simulink model "TV_Rev2_DynTest_SIMULINK"  (R2021a)
settings: Solver=FixedStepAuto  StartTime=0.0  StopTime=40  FixedStep=0.01  RelTol=1e-3
values from neighbouring files (symbols this model uses):
  Delta11T = xlsread('TV Dynamic Test data_EXCEL.xlsx', 'Steering','L2:L55' )    [TorqueVectoring_Rev2_Parameters_MATLAB.m]
  Delta12T = xlsread('TV Dynamic Test data_EXCEL.xlsx', 'Steering','M2:M55' )    [TorqueVectoring_Rev2_Parameters_MATLAB.m]
  DeltaT = xlsread('TV Dynamic Test data_EXCEL.xlsx', 'Steering','K2:K55' )    [TorqueVectoring_Rev2_Parameters_MATLAB.m]
  Tmaxf = 250    [TorqueVectoring_Rev2_Parameters_MATLAB.m]
  Tmaxr = 250    [TorqueVectoring_Rev2_Parameters_MATLAB.m]
undefined symbols (not defined in the file or in its folder): sigbuilder_block
libraries: simulink_extras x2
settings Model: Creator=CptBrownPants  LastModifiedBy=Pickett
settings SolverCC: AlgebraicLoopSolver=TrustRegion
settings OptimizationCC: DefaultParameterBehavior=Inlined  EnhancedBackFolding=on  PassReuseOutputArgsAs=Individual arguments  ZeroExternalMemoryAtStartup=off  ZeroInternalMemoryAtStartup=off  InitFltsAndDblsToZero=on  MaxStackSize=2048  OptimizeBlockOrder=speed  DifferentSizesBufferReuse=on  OptimizationCustomize=off  EfficientTunableParamExpr=on
settings DebuggingCC: ParameterTunabilityLossMsg=error  SFMachineParentedDataDiag=warning
settings HardwareCC: ProdBitPerPointer=32  ProdBitPerSizeT=32  ProdBitPerPtrDiffT=32  ProdLargestAtomicInteger=Long  ProdLargestAtomicFloat=Double  ProdEndianess=BigEndian  ProdWordSize=32  ProdHWDeviceType=Freescale->32-bit PowerPC
settings SFSimCC: MATLABDynamicMemAlloc=off
settings RTWCC: Description=Create UserLibraries for MoTeC M1 Build  SystemTargetFile=MoTeC.tlc  GenCodeOnly=on  TemplateMakefile=MoTeCUserlibMakefile.tmf  PostCodeGenCommand=MoTeCUtil.m1_post_process(buildInfo)
settings CodeAppCC: ForceParamTrailComments=on  IgnoreCustomStorageClasses=off  OperatorAnnotations=on  SimulinkDataObjDesc=on  SFDataObjDesc=on  InsertBlockDesc=on
settings STFCustomTargetCC: TargetLangStandard=C99 (ISO)  MultiwordLength=256  GenerateSampleERTMain=on  CombineOutputUpdateFcns=on  ERTCustomFileBanners=on  SupportContinuousTime=off  SupportNonInlinedSFcns=off  RemoveResetFunc=on  MATLABClassNameForMDSCustomization=Simulink.SoftwareTarget.ERTCustomization  GRTInterface=off  UseToolchainInfoCompliant=off  SystemTargetFile=MoTeC.tlc
settings ERTTargetCC: TargetLangStandard=C99 (ISO)  GenerateSampleERTMain=on  ParMdlRefBuildCompliant=off  CompOptLevelCompliant=off  ConcurrentExecutionCompliant=off  ModelStepFunctionPrototypeControlCompliant=off  CPPClassGenCompliant=off  UseToolchainInfoCompliant=off  InlinedParameterPlacement=NonHierarchical  ERTCustomFileTemplate=MoTeCFileProcess.tlc  EnableUserReplacementTypes=on

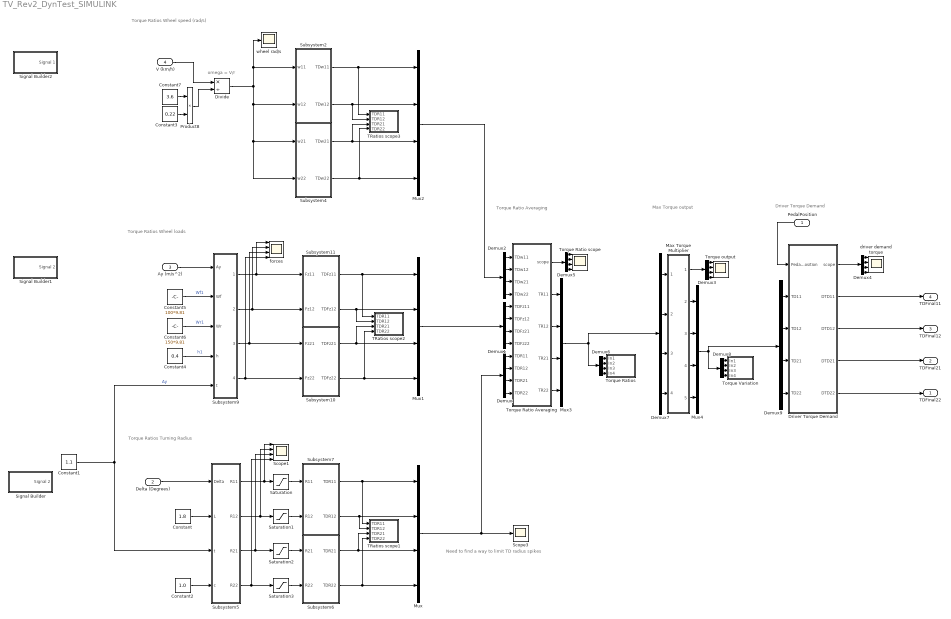
== system TV_Rev2_DynTest_SIMULINK ==
  note: Driver Torque Demand
  note: Max Torque output
  note: Torque Ratio Averaging
  note: Need to find a way to limit TD radius spikes
  note: Torque Ratios Wheel speed (rad/s)
  note: Torque Ratios Wheel loads
  note: Torque Ratios Turning Radius
  note: omega = V/r
  PedalPosition : Inport
  Delta (Degrees) : Inport  Port=2
  Ay (m/s^2) : Inport  Port=3
  V (km/h) : Inport  Port=4
  Constant : Constant  Value=1.8
  Constant1 : Constant  Value=1.1
  Constant2 : Constant  Value=1.0
  Constant3 : Constant  Value=0.22
  Constant4 : Constant  Value=0.4
  Constant5 : Constant  Value=100*9.81
  Constant6 : Constant  Value=150*9.81
  Constant7 : Constant  Value=3.6
  Demux{,1..9} (10 alike) : Demux
  Divide : Product  Inputs=*/
  Driver Torque Demand : Subsystem
  Max Torque Multiplier : Subsystem
  Mux{,1..4} (5 alike) : Mux
  Product8 : Product
  Saturation{,1..3} (4 alike) : Saturate  UpperLimit=100  LowerLimit=-100
  Scope1 : Scope  NumInputPorts=4
  Scope3 : Scope
  Signal Builder : Subsystem  Tag=STV Subsys  LoadFcn=sigbuilder_block('load');  StartFcn=sigbuilder_block('start');  StopFcn=sigbuilder_block('stop');  ClipboardFcn=sigbuilder_block('clipboard');  mask(Sigbuilder block){tuvar=[0:10]}
      mask help: Simulink:masks:SigbuilderBlock_MD
      mask init:
      | if ~strcmp(get_param(bdroot(gcbh),'SimulationStatus'),'stopped') tuvar = sigbuilder_block('maskInit'); end
      settings: CopyFcn=sigbuilder_block('copy');  DeleteFcn=sigbuilder_block('delete');  ModelCloseFcn=sigbuilder_block('modelClose');  PreSaveFcn=sigbuilder_block('preSave');  PauseFcn=sigbuilder_block('pause');  ContinueFcn=sigbuilder_block('continue');  NameChangeFcn=sigbuilder_block('namechange');  OpenFcn=sigbuilder_block('open',[143 201 550 400 ]);  CloseFcn=sigbuilder_block('close');
      mask Display: plot(0, 0, 100, 100,[2, 2, 32, 32, 2], [68, 8, 8, 68, 68],[32, 2], [38, 38], [32, 19, 2],[53, 60, 44], [32, 17, 17, 2],[16, 16, 31, 31]);txt = getActiveGroup(gcbh);text(2, 100, txt,'verticalAlignment', 'top');
  Signal Builder1 : Subsystem  Tag=STV Subsys  LoadFcn=sigbuilder_block('load');  StartFcn=sigbuilder_block('start');  StopFcn=sigbuilder_block('stop');  ClipboardFcn=sigbuilder_block('clipboard');  mask(Sigbuilder block){tuvar=[0:10]}
      mask help: Simulink:masks:SigbuilderBlock_MD
      mask init:
      | if ~strcmp(get_param(bdroot(gcbh),'SimulationStatus'),'stopped') tuvar = sigbuilder_block('maskInit'); end
      settings: CopyFcn=sigbuilder_block('copy');  DeleteFcn=sigbuilder_block('delete');  ModelCloseFcn=sigbuilder_block('modelClose');  PreSaveFcn=sigbuilder_block('preSave');  PauseFcn=sigbuilder_block('pause');  ContinueFcn=sigbuilder_block('continue');  NameChangeFcn=sigbuilder_block('namechange');  OpenFcn=sigbuilder_block('open',[437.6 199.2 550.4 400 ]);  CloseFcn=sigbuilder_block('close');
      mask Display: plot(0, 0, 100, 100,[2, 2, 32, 32, 2], [68, 8, 8, 68, 68],[32, 2], [38, 38], [32, 19, 2],[53, 60, 44], [32, 17, 17, 2],[16, 16, 31, 31]);txt = getActiveGroup(gcbh);text(2, 100, txt,'verticalAlignment', 'top');
  Signal Builder2 : Subsystem  Tag=STV Subsys  LoadFcn=sigbuilder_block('load');  StartFcn=sigbuilder_block('start');  StopFcn=sigbuilder_block('stop');  ClipboardFcn=sigbuilder_block('clipboard');  mask(Sigbuilder block){tuvar=[0:10]}
      mask help: Simulink:masks:SigbuilderBlock_MD
      mask init:
      | if ~strcmp(get_param(bdroot(gcbh),'SimulationStatus'),'stopped') tuvar = sigbuilder_block('maskInit'); end
      settings: CopyFcn=sigbuilder_block('copy');  DeleteFcn=sigbuilder_block('delete');  ModelCloseFcn=sigbuilder_block('modelClose');  PreSaveFcn=sigbuilder_block('preSave');  PauseFcn=sigbuilder_block('pause');  ContinueFcn=sigbuilder_block('continue');  NameChangeFcn=sigbuilder_block('namechange');  OpenFcn=sigbuilder_block('open',[437.6 199.2 550.4 400 ]);  CloseFcn=sigbuilder_block('close');
      mask Display: plot(0, 0, 100, 100,[2, 2, 32, 32, 2], [68, 8, 8, 68, 68],[32, 2], [38, 38], [32, 19, 2],[53, 60, 44], [32, 17, 17, 2],[16, 16, 31, 31]);txt = getActiveGroup(gcbh);text(2, 100, txt,'verticalAlignment', 'top');
  Subsystem10 : Subsystem
  Subsystem11 : Subsystem
  Subsystem2 : Subsystem
  Subsystem4 : Subsystem
  Subsystem5 : Subsystem
  Subsystem6 : Subsystem
  Subsystem7 : Subsystem
  Subsystem9 : Subsystem
  TRatios scope1 : Subsystem
  TRatios scope2 : Subsystem
  TRatios scope3 : Subsystem
  Torque Ratio Averaging : Subsystem
  Torque Ratio scope : Scope  NumInputPorts=4
  "Torque Ratios " : Subsystem
  Torque Variation : Subsystem
  Torque output : Scope  NumInputPorts=4
  driver demand torque : Scope  NumInputPorts=4
  forces : Scope  NumInputPorts=4
  wheel rad/s : Scope
  TDFinal22 : Outport
  TDFinal21 : Outport  Port=2
  TDFinal12 : Outport  Port=3
  TDFinal11 : Outport  Port=4
  wires:
  Subsystem2/2(TDw12) -> Mux2/2, TRatios scope3/2(TDR12)
  Subsystem2/1(TDw11) -> Mux2/1, TRatios scope3/1(TDR11)
  Subsystem4/2(TDw22) -> Mux2/4, TRatios scope3/4(TDR22)
  Subsystem4/1(TDw21) -> Mux2/3, TRatios scope3/3(TDR21)
  Subsystem7/2(TDR12) -> Mux/2, TRatios scope1/2(TDR12)
  Subsystem7/1(TDR11) -> Mux/1, TRatios scope1/1(TDR11)
  Subsystem6/2(TDR22) -> Mux/4, TRatios scope1/4(TDR22)
  Subsystem6/1(TDR21) -> Mux/3, TRatios scope1/3(TDR21)
  Subsystem5/1(R11) -> Scope1/1, Saturation/1
  Saturation/1 -> Subsystem7/1(R11)
  Subsystem5/2(R12) -> Scope1/2, Saturation1/1
  Subsystem5/4(R22) -> Saturation3/1, Scope1/4
  Subsystem5/3(R21) -> Saturation2/1, Scope1/3
  Constant1/1 -> Subsystem5/3(t), Subsystem9/5(t)  "Ay"
  Constant/1 -> Subsystem5/2(L)
  Saturation1/1 -> Subsystem7/2(R12)
  Constant2/1 -> Subsystem5/4(c)
  Saturation2/1 -> Subsystem6/1(R21)
  Saturation3/1 -> Subsystem6/2(R22)
  Subsystem9/2(Fz12) -> forces/2, Subsystem11/2(Fz12)
  Subsystem9/3(Fz21) -> forces/3, Subsystem10/1(Fz21)
  Constant4/1 -> Subsystem9/4(h)  "h1"
  Subsystem9/1(Fz11) -> Subsystem11/1(Fz11), forces/1
  Constant6/1 -> Subsystem9/3(Wr)  "Wr1"
  Subsystem9/4(Fz22) -> Subsystem10/2(Fz22), forces/4
  Constant5/1 -> Subsystem9/2(Wf)  "Wf1"
  Divide/1 -> wheel rad/s/1, Subsystem2/1(w11), Subsystem4/2(w22), Subsystem4/1(w21), Subsystem2/2(w12)
  Constant3/1 -> Product8/2
  Constant7/1 -> Product8/1
  Product8/1 -> Divide/2
  Mux/1 -> Demux/1, Scope3/1
  Demux/1 -> Torque Ratio Averaging/9(TDR11)
  Demux/2 -> Torque Ratio Averaging/10(TDR12)
  Demux/3 -> Torque Ratio Averaging/11(TDR21)
  Demux/4 -> Torque Ratio Averaging/12(TDR22)
  Subsystem10/1(TDFz21) -> Mux1/3, TRatios scope2/3(TDR21)
  Subsystem10/2(TDFz22) -> Mux1/4, TRatios scope2/4(TDR22)
  Subsystem11/2(TDFz12) -> Mux1/2, TRatios scope2/2(TDR12)
  Subsystem11/1(TDFz11) -> Mux1/1, TRatios scope2/1(TDR11)
  Demux1/1 -> Torque Ratio Averaging/5(TDFz11)
  Demux1/2 -> Torque Ratio Averaging/6(TDFz12)
  Demux1/3 -> Torque Ratio Averaging/7(TDFz21)
  Demux1/4 -> Torque Ratio Averaging/8(TDFz22)
  Mux1/1 -> Demux1/1
  Demux2/1 -> Torque Ratio Averaging/1(TDw11)
  Demux2/2 -> Torque Ratio Averaging/2(TDw12)
  Demux2/3 -> Torque Ratio Averaging/3(TDw21)
  Demux2/4 -> Torque Ratio Averaging/4(TDw22)
  Mux2/1 -> Demux2/1
  Demux3/2 -> Torque output/2
  Demux3/3 -> Torque output/3
  Demux3/4 -> Torque output/4
  Demux3/1 -> Torque output/1
  Demux4/1 -> driver demand torque/1
  Demux4/2 -> driver demand torque/2
  Demux4/3 -> driver demand torque/3
  Demux4/4 -> driver demand torque/4
  Driver Torque Demand/2(DTD11) -> TDFinal11/1
  Driver Torque Demand/3(DTD12) -> TDFinal12/1
  Driver Torque Demand/4(DTD21) -> TDFinal21/1
  Driver Torque Demand/5(DTD22) -> TDFinal22/1
  Max Torque Multiplier/1(scope) -> Demux3/1
  Driver Torque Demand/1(scope) -> Demux4/1
  Demux5/1 -> Torque Ratio scope/1
  Demux5/4 -> Torque Ratio scope/4
  Demux5/3 -> Torque Ratio scope/3
  Demux5/2 -> Torque Ratio scope/2
  Torque Ratio Averaging/1(scope) -> Demux5/1
  Torque Ratio Averaging/2(TR11) -> Mux3/1
  Torque Ratio Averaging/3(TR12) -> Mux3/2
  Torque Ratio Averaging/4(TR21) -> Mux3/3
  Torque Ratio Averaging/5(TR22) -> Mux3/4
  Demux6/3 -> "Torque Ratios "/3(In3)
  Demux6/1 -> "Torque Ratios "/1(In1)
  Demux6/2 -> "Torque Ratios "/2(In2)
  Demux6/4 -> "Torque Ratios "/4(In4)
  Mux3/1 -> Demux7/1, Demux6/1
  Demux7/1 -> Max Torque Multiplier/1(TR11)
  Demux7/2 -> Max Torque Multiplier/2(TR12)
  Demux7/3 -> Max Torque Multiplier/3(TR21)
  Demux7/4 -> Max Torque Multiplier/4(TR22)
  Max Torque Multiplier/2(TD11) -> Mux4/1
  Max Torque Multiplier/3(TD12) -> Mux4/2
  Max Torque Multiplier/4(TD21) -> Mux4/3
  Max Torque Multiplier/5(TD22) -> Mux4/4
  Demux8/4 -> Torque Variation/4(In4)
  Demux8/2 -> Torque Variation/2(In2)
  Demux8/1 -> Torque Variation/1(In1)
  Demux8/3 -> Torque Variation/3(In3)
  Mux4/1 -> Demux9/1, Demux8/1
  Demux9/1 -> Driver Torque Demand/2(TD11)
  Demux9/2 -> Driver Torque Demand/3(TD12)
  Demux9/3 -> Driver Torque Demand/4(TD21)
  Demux9/4 -> Driver Torque Demand/5(TD22)
  Delta (Degrees)/1 -> Subsystem5/1(Delta)
  Ay (m/s^2)/1 -> Subsystem9/1(Ay)
  V (km/h)/1 -> Divide/1
  PedalPosition/1 -> Driver Torque Demand/1(PedalPosition)

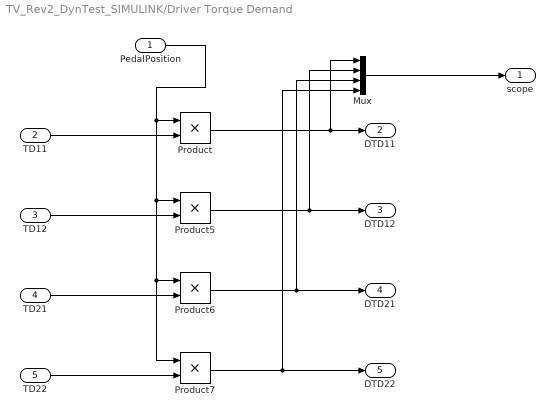
== system TV_Rev2_DynTest_SIMULINK/Driver Torque Demand ==
  PedalPosition : Inport
  TD11 : Inport  Port=2
  TD12 : Inport  Port=3
  TD21 : Inport  Port=4
  TD22 : Inport  Port=5
  Mux : Mux
  Product{,5..7} (4 alike) : Product
  scope : Outport
  DTD11 : Outport  Port=2
  DTD12 : Outport  Port=3
  DTD21 : Outport  Port=4
  DTD22 : Outport  Port=5
  wires:
  TD22/1 -> Product7/2
  PedalPosition/1 -> Product7/1, Product6/1, Product5/1, Product/1
  TD11/1 -> Product/2
  TD21/1 -> Product6/2
  TD12/1 -> Product5/2
  Product/1 -> Mux/1, DTD11/1
  Product6/1 -> Mux/3, DTD21/1
  Product5/1 -> Mux/2, DTD12/1
  Mux/1 -> scope/1
  Product7/1 -> Mux/4, DTD22/1

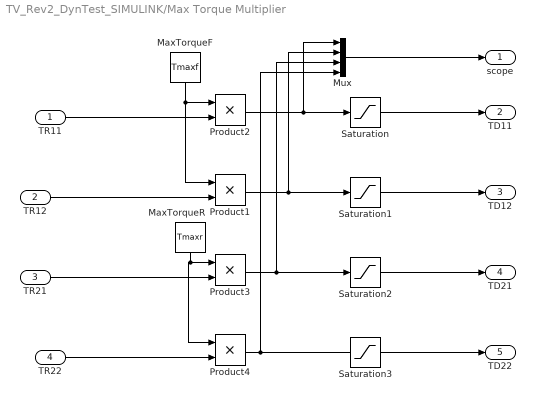
== system TV_Rev2_DynTest_SIMULINK/Max Torque Multiplier ==
  TR11 : Inport
  TR12 : Inport  Port=2
  TR21 : Inport  Port=3
  TR22 : Inport  Port=4
  MaxTorqueF : Constant  Value=Tmaxf
  MaxTorqueR : Constant  Value=Tmaxr
  Mux : Mux
  Product{1..4} (4 alike) : Product
  Saturation{,1..3} (4 alike) : Saturate  UpperLimit=250  LowerLimit=-250
  scope : Outport
  TD11 : Outport  Port=2
  TD12 : Outport  Port=3
  TD21 : Outport  Port=4
  TD22 : Outport  Port=5
  wires:
  Product3/1 -> Mux/3, Saturation2/1
  MaxTorqueR/1 -> Product4/1, Product3/1
  MaxTorqueF/1 -> Product1/1, Product2/1
  TR22/1 -> Product4/2
  TR11/1 -> Product2/2
  TR12/1 -> Product1/2
  Product1/1 -> Mux/2, Saturation1/1
  Product4/1 -> Mux/4, TD22/1
  Product2/1 -> Mux/1, Saturation/1
  TR21/1 -> Product3/2
  Mux/1 -> scope/1
  Saturation/1 -> TD11/1
  Saturation1/1 -> TD12/1
  Saturation2/1 -> TD21/1

== system TV_Rev2_DynTest_SIMULINK/Signal Builder ==
  Demux : Demux  Tag=STV Demux  Outputs=1
      settings: DisplayOption=none
  FromWs : FromWorkspace  Tag=STV FromWs  VariableName=tuvar
      SigBuilderData=|
      | common.afterFinalStr = 'Extrapolate'
      | common.sampleTime = 0
      | dataSet.timeRange = [0 50]
      | dataSet.name = 'Group 1'
      | sbobj.Groups.Name = 'Group 1'
      | sbobj.Groups.Signals.Name = 'Signal 2'
      | sbobj.Groups.Signals.XData = [0 0.25 0.5 0.75 1 1.25 1.5 1.75 2 2.25 2.5 2.75 3 3.25 3.5 3.75 4 4.25 4.5 4.75 5 5.25 5.5 5.75 6 6.25 6.5 6.75 7 7.25 7.5 7.75 8 8.25 8.5 8.75 9 9.25 9.5 9.75 10 10.25 10.5 10.75 11 11.25 11.5 11.75 12 12.25 12.5 12.75 13 13.25 13.5 13.75 14 14.25 14.5 14.75 15 15.25 15.5 15.75 16 16.25 16.5 16.75 17 17.25 17.5 17.75 18 18.25 18.5 18.75 19 19.25 19.5 19.75 20 20.25 20.5 20.75 21 21.25 21.5 21.75 22 22.25 22.5 22.75 23 23.25 23.5 23.75 24 24.25 24.5 24.75 25 25.25 25.5 25.75 26 26.25 26.5 26.75 27 27.25 27.5 27.75 28 28.25 28.5 28.75 29 29.25 29.5 29.75 30 30.25 30.5 30.75 31 31.25 31.5 31.75 32 32.25 32.5 32.75 33 33.25 33.5 33.75 34 34.25 34.5 34.75 35 35.25 35.5 35.75 36 36.25 36.5 36.75 37 37.25 37.5 37.75 38 38.25 38.5 38.75 39 39.25 39.5 39.75 50]
      | sbobj.Groups.Signals.YData = [50.001 50.001 50.001 50.001 50.001 50.001 50.001 50.001 50.001 50.001 50.001 50.001 50.001 50.001 50.001 50.001 50.001 50.001 50.001 50.001 50.001 49 48 47 46 45 44 43 42 41 40 39 38 37 36 35 34 33 32 31 30 31 32 33 34 35 36 37 38 39 40 41 42 43 44 45 46 47 48 49 50.001 51 52 53 54 55 56 57 58 59 60 61 62 63 64 65 66 67 68 69 70 69 68 67 66 65 64 63 62 61 60 59 58 57 56 55 54 53 52 51 50.001 49 48 47 46 45 44 43 42 41 40 39 38 37 36 35 34 33 32 31 30 31 32 33 34 35 36 37 38 39 40 41 42 43 44 45 46 47 48 49 50.001 50.001 50.001 50.001 50.001 50.001 50.001 50.001 50.001 50.001 50.001 50.001 50.001 50.001 50.001 50.001 50.001 50.001 50.001 50.001 50.001]
      | sbobj.Groups.TimeRange = [0 50]
  Signal 2 : Outport  Tag=STV Outport
  wires:
  FromWs/1 -> Demux/1
  Demux/1 -> Signal 2/1

== system TV_Rev2_DynTest_SIMULINK/Signal Builder1 ==
  Demux : Demux  Tag=STV Demux  Outputs=1
      settings: DisplayOption=none
  FromWs : FromWorkspace  Tag=STV FromWs  VariableName=tuvar
      SigBuilderData=|
      | common.afterFinalStr = 'Extrapolate'
      | common.sampleTime = 0
      | dataSet.timeRange = [0 50]
      | dataSet.name = 'Group 1'
      | sbobj.Groups.Name = 'Group 1'
      | sbobj.Groups.Signals.Name = 'Signal 2'
      | sbobj.Groups.Signals.XData = [0 0.25 0.5 0.75 1 1.25 1.5 1.75 2 2.25 2.5 2.75 3 3.25 3.5 3.75 4 4.25 4.5 4.75 5 5.25 5.5 5.75 6 6.25 6.5 6.75 7 7.25 7.5 7.75 8 8.25 8.5 8.75 9 9.25 9.5 9.75 10 10.25 10.5 10.75 11 11.25 11.5 11.75 12 12.25 12.5 12.75 13 13.25 13.5 13.75 14 14.25 14.5 14.75 15 15.25 15.5 15.75 16 16.25 16.5 16.75 17 17.25 17.5 17.75 18 18.25 18.5 18.75 19 19.25 19.5 19.75 20 20.25 20.5 20.75 21 21.25 21.5 21.75 22 22.25 22.5 22.75 23 23.25 23.5 23.75 24 24.25 24.5 24.75 25 25.25 25.5 25.75 26 26.25 26.5 26.75 27 27.25 27.5 27.75 28 28.25 28.5 28.75 29 29.25 29.5 29.75 30 30.25 30.5 30.75 31 31.25 31.5 31.75 32 32.25 32.5 32.75 33 33.25 33.5 33.75 34 34.25 34.5 34.75 35 35.25 35.5 35.75 36 36.25 36.5 36.75 37 37.25 37.5 37.75 38 38.25 38.5 38.75 39 39.25 39.5 39.75 40 50]
      | sbobj.Groups.Signals.YData = [0 1.37326168587e-07 5.49304674348e-07 1.23593551728e-06 2.19721869739e-06 3.43315421468e-06 4.94374206914e-06 6.72898226077e-06 8.78887478957e-06 1.11234196556e-05 1.37326168587e-05 1.6616466399e-05 ... (162 elements, 1x162)]
      | sbobj.Groups.TimeRange = [0 50]
  Signal 2 : Outport  Tag=STV Outport
  wires:
  FromWs/1 -> Demux/1
  Demux/1 -> Signal 2/1

== system TV_Rev2_DynTest_SIMULINK/Signal Builder2 ==
  Demux : Demux  Tag=STV Demux  Outputs=1
      settings: DisplayOption=none
  FromWs : FromWorkspace  Tag=STV FromWs  VariableName=tuvar
      SigBuilderData=|
      | common.afterFinalStr = 'Extrapolate'
      | common.sampleTime = 0
      | dataSet.timeRange = [0 50]
      | dataSet.name = 'Group 1'
      | sbobj.Groups.Name = 'Group 1'
      | sbobj.Groups.Signals.Name = 'Signal 1'
      | sbobj.Groups.Signals.XData = [0 0.25 0.5 0.75 1 1.25 1.5 1.75 2 2.25 2.5 2.75 3 3.25 3.5 3.75 4 4.25 4.5 4.75 5 5.25 5.5 5.75 6 6.25 6.5 6.75 7 7.25 7.5 7.75 8 8.25 8.5 8.75 9 9.25 9.5 9.75 10 10.25 10.5 10.75 11 11.25 11.5 11.75 12 12.25 12.5 12.75 13 13.25 13.5 13.75 14 14.25 14.5 14.75 15 15.25 15.5 15.75 16 16.25 16.5 16.75 17 17.25 17.5 17.75 18 18.25 18.5 18.75 19 19.25 19.5 19.75 20 20.25 20.5 20.75 21 21.25 21.5 21.75 22 22.25 22.5 22.75 23 23.25 23.5 23.75 24 24.25 24.5 24.75 25 25.25 25.5 25.75 26 26.25 26.5 26.75 27 27.25 27.5 27.75 28 28.25 28.5 28.75 29 29.25 29.5 29.75 30 30.25 30.5 30.75 31 31.25 31.5 31.75 32 32.25 32.5 32.75 33 33.25 33.5 33.75 34 34.25 34.5 34.75 35 35.25 35.5 35.75 36 36.25 36.5 36.75 37 37.25 37.5 37.75 38 38.25 38.5 38.75 39 39.25 39.5 39.75 40 50]
      | sbobj.Groups.Signals.YData = [0 3 6 9 12 15 18 21 24 27 30 33 36 39 42 45 48 51 54 57 60 60 60 60 60 60 60 60 60 60 60 60 60 60 60 60 60 60 60 60 60 60 60 60 60 60 60 60 60 60 60 60 60 60 60 60 60 60 60 60 60 60 60 60 60 60 60 60 60 60 60 60 60 60 60 60 60 60 60 60 60 60 60 60 60 60 60 60 60 60 60 60 60 60 60 60 60 60 60 60 60 60 60 60 60 60 60 60 60 60 60 60 60 60 60 60 60 60 60 60 60 60 60 60 60 60 60 60 60 60 60 60 60 60 60 60 60 60 60 60 60 57 54 51 48 45 42 39 36 33 30 27 24 21 18 15 12 9 6 3 0 0]
      | sbobj.Groups.TimeRange = [0 50]
  Signal 1 : Outport  Tag=STV Outport
  wires:
  FromWs/1 -> Demux/1
  Demux/1 -> Signal 1/1

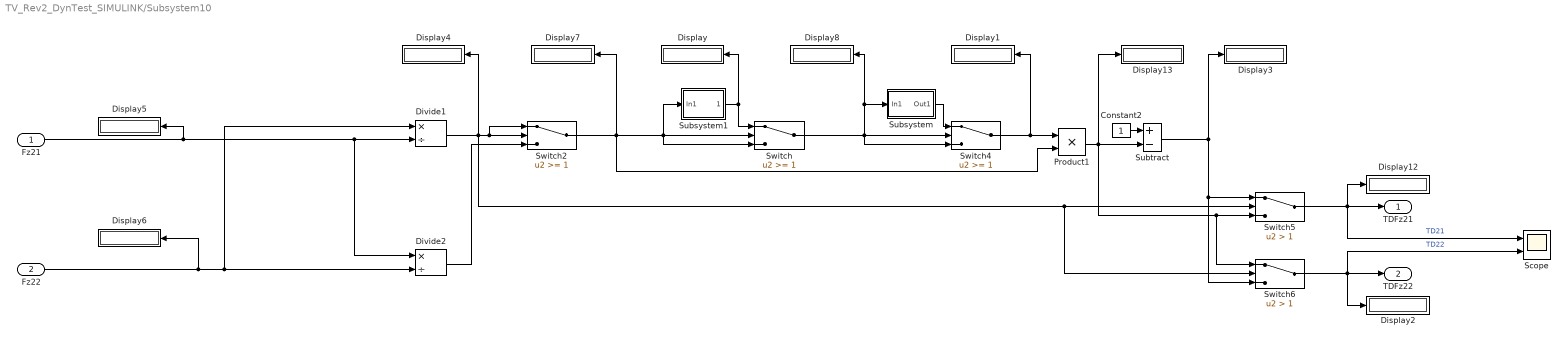
== system TV_Rev2_DynTest_SIMULINK/Subsystem10 ==
  Fz21 : Inport
  Fz22 : Inport  Port=2
  Constant2 : Constant
  Display{,1..8,12..13} (11 alike) : Display
  Divide1 : Product  Inputs=*/
  Divide2 : Product  Inputs=*/
  Product1 : Product
  Scope : Scope  NumInputPorts=2
  Subsystem : Subsystem
  Subsystem1 : Subsystem
  Subtract : Sum  Inputs=+-
  Switch : Switch  Threshold=1
  Switch2 : Switch  Threshold=1
  Switch4 : Switch  Threshold=1
  Switch5 : Switch  Criteria=u2 > Threshold  Threshold=1
  Switch6 : Switch  Criteria=u2 > Threshold  Threshold=1
  TDFz21 : Outport
  TDFz22 : Outport  Port=2
  wires:
  Switch6/1 -> Scope/2, Display2/1, TDFz22/1  "TD22"
  Fz21/1 -> Display5/1, Divide2/1, Divide1/2
  Switch5/1 -> TDFz21/1, Scope/1, Display12/1  "TD21"
  Subsystem/1(Out1) -> Switch4/1
  Switch/1 -> Switch4/3, Switch4/2, Display8/1, Subsystem/1(In1)
  Switch2/1 -> Product1/2, Display7/1, Switch/2, Switch/3, Subsystem1/1(In1)
  Subsystem1/1(Out1) -> Switch/1, Display/1
  Constant2/1 -> Subtract/1
  Subtract/1 -> Display3/1, Switch6/3, Switch5/1
  Product1/1 -> Switch6/1, Switch5/3, Display13/1, Subtract/2
  Divide2/1 -> Switch2/3
  Switch4/1 -> Product1/1, Display1/1
  Divide1/1 -> Switch6/2, Switch5/2, Display4/1, Switch2/1, Switch2/2
  Fz22/1 -> Display6/1, Divide1/1, Divide2/2

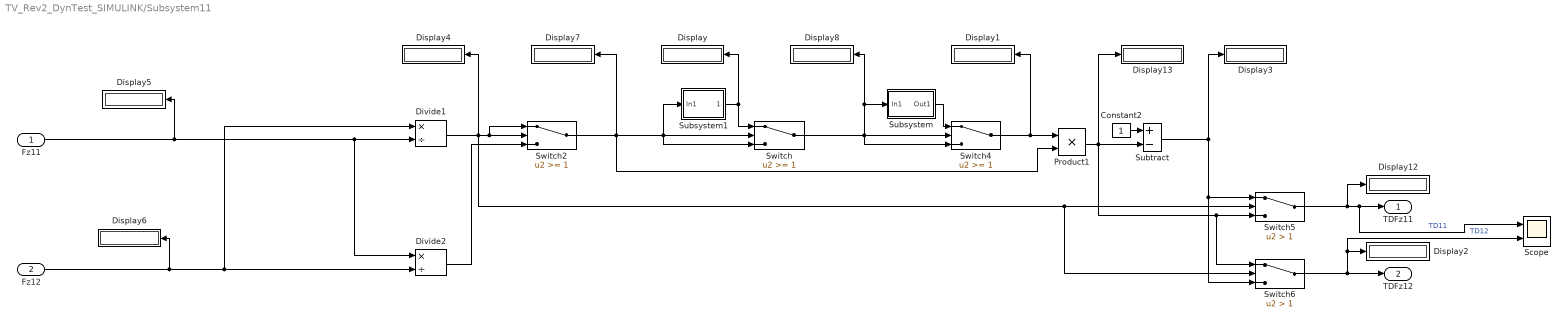
== system TV_Rev2_DynTest_SIMULINK/Subsystem11 ==
  Fz11 : Inport
  Fz12 : Inport  Port=2
  Constant2 : Constant
  Display{,1..8,12..13} (11 alike) : Display
  Divide1 : Product  Inputs=*/
  Divide2 : Product  Inputs=*/
  Product1 : Product
  Scope : Scope  NumInputPorts=2
  Subsystem : Subsystem
  Subsystem1 : Subsystem
  Subtract : Sum  Inputs=+-
  Switch : Switch  Threshold=1
  Switch2 : Switch  Threshold=1
  Switch4 : Switch  Threshold=1
  Switch5 : Switch  Criteria=u2 > Threshold  Threshold=1
  Switch6 : Switch  Criteria=u2 > Threshold  Threshold=1
  TDFz11 : Outport
  TDFz12 : Outport  Port=2
  wires:
  Switch6/1 -> Scope/2, Display2/1, TDFz12/1  "TD12"
  Fz11/1 -> Display5/1, Divide2/1, Divide1/2
  Switch5/1 -> Display12/1, Scope/1, TDFz11/1  "TD11"
  Subsystem/1(Out1) -> Switch4/1
  Switch/1 -> Switch4/3, Switch4/2, Display8/1, Subsystem/1(In1)
  Switch2/1 -> Product1/2, Display7/1, Switch/2, Switch/3, Subsystem1/1(In1)
  Subsystem1/1(Out1) -> Switch/1, Display/1
  Constant2/1 -> Subtract/1
  Subtract/1 -> Display3/1, Switch6/3, Switch5/1
  Product1/1 -> Switch6/1, Switch5/3, Display13/1, Subtract/2
  Divide2/1 -> Switch2/3
  Switch4/1 -> Product1/1, Display1/1
  Divide1/1 -> Switch6/2, Switch5/2, Display4/1, Switch2/1, Switch2/2
  Fz12/1 -> Display6/1, Divide1/1, Divide2/2

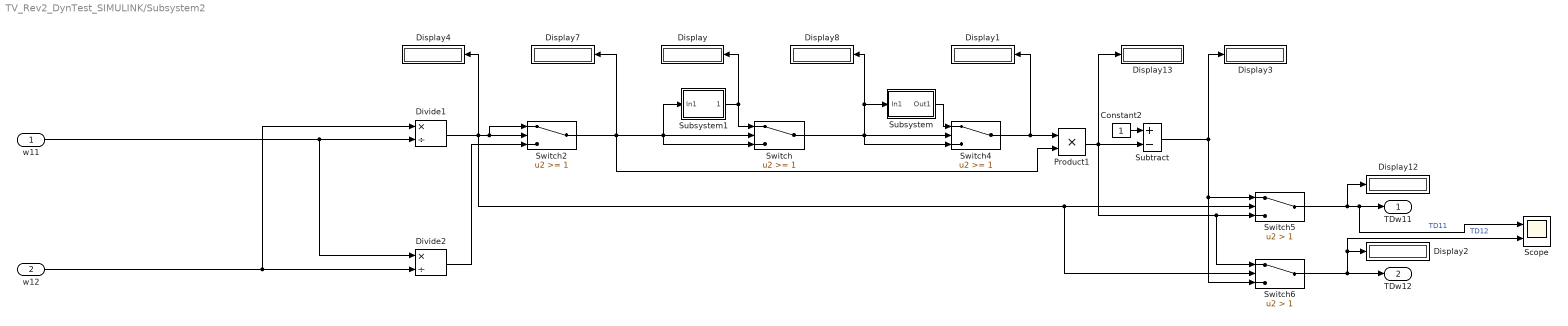
== system TV_Rev2_DynTest_SIMULINK/Subsystem2 ==
  w11 : Inport
  w12 : Inport  Port=2
  Constant2 : Constant
  Display{,1..4,7..8,12..13} (9 alike) : Display
  Divide1 : Product  Inputs=*/
  Divide2 : Product  Inputs=*/
  Product1 : Product
  Scope : Scope  NumInputPorts=2
  Subsystem : Subsystem
  Subsystem1 : Subsystem
  Subtract : Sum  Inputs=+-
  Switch : Switch  Threshold=1
  Switch2 : Switch  Threshold=1
  Switch4 : Switch  Threshold=1
  Switch5 : Switch  Criteria=u2 > Threshold  Threshold=1
  Switch6 : Switch  Criteria=u2 > Threshold  Threshold=1
  TDw11 : Outport
  TDw12 : Outport  Port=2
  wires:
  Divide1/1 -> Switch2/2, Switch2/1, Display4/1, Switch5/2, Switch6/2
  Switch4/1 -> Display1/1, Product1/1
  Divide2/1 -> Switch2/3
  Product1/1 -> Subtract/2, Display13/1, Switch5/3, Switch6/1
  Subtract/1 -> Switch5/1, Switch6/3, Display3/1
  Constant2/1 -> Subtract/1
  Subsystem1/1(Out1) -> Display/1, Switch/1
  Switch2/1 -> Subsystem1/1(In1), Switch/3, Switch/2, Display7/1, Product1/2
  Switch/1 -> Subsystem/1(In1), Display8/1, Switch4/2, Switch4/3
  Subsystem/1(Out1) -> Switch4/1
  Switch5/1 -> TDw11/1, Scope/1, Display12/1  "TD11"
  Switch6/1 -> TDw12/1, Display2/1, Scope/2  "TD12"
  w11/1 -> Divide2/1, Divide1/2
  w12/1 -> Divide1/1, Divide2/2

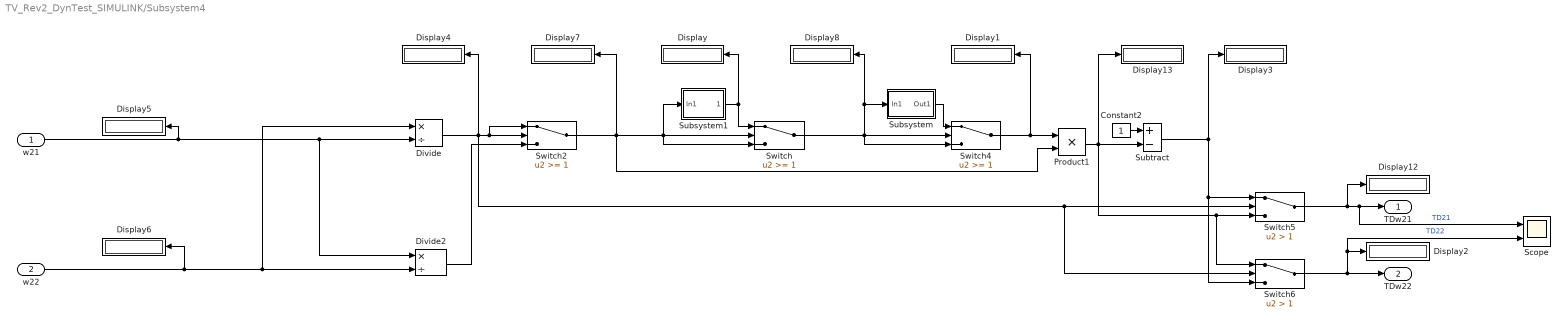
== system TV_Rev2_DynTest_SIMULINK/Subsystem4 ==
  w21 : Inport
  w22 : Inport  Port=2
  Constant2 : Constant
  Display{,1..8,12..13} (11 alike) : Display
  Divide : Product  Inputs=*/
  Divide2 : Product  Inputs=*/
  Product1 : Product
  Scope : Scope  NumInputPorts=2
  Subsystem : Subsystem
  Subsystem1 : Subsystem
  Subtract : Sum  Inputs=+-
  Switch : Switch  Threshold=1
  Switch2 : Switch  Threshold=1
  Switch4 : Switch  Threshold=1
  Switch5 : Switch  Criteria=u2 > Threshold  Threshold=1
  Switch6 : Switch  Criteria=u2 > Threshold  Threshold=1
  TDw21 : Outport
  TDw22 : Outport  Port=2
  wires:
  Divide/1 -> Switch2/2, Switch2/1, Display4/1, Switch5/2, Switch6/2
  Switch4/1 -> Display1/1, Product1/1
  Divide2/1 -> Switch2/3
  Product1/1 -> Subtract/2, Display13/1, Switch5/3, Switch6/1
  Subtract/1 -> Switch5/1, Switch6/3, Display3/1
  Constant2/1 -> Subtract/1
  Subsystem1/1(Out1) -> Display/1, Switch/1
  Switch2/1 -> Subsystem1/1(In1), Switch/3, Switch/2, Display7/1, Product1/2
  Switch/1 -> Subsystem/1(In1), Display8/1, Switch4/2, Switch4/3
  Subsystem/1(Out1) -> Switch4/1
  Switch5/1 -> TDw21/1, Scope/1, Display12/1  "TD21"
  Switch6/1 -> TDw22/1, Display2/1, Scope/2  "TD22"
  w21/1 -> Display5/1, Divide/2, Divide2/1
  w22/1 -> Display6/1, Divide/1, Divide2/2

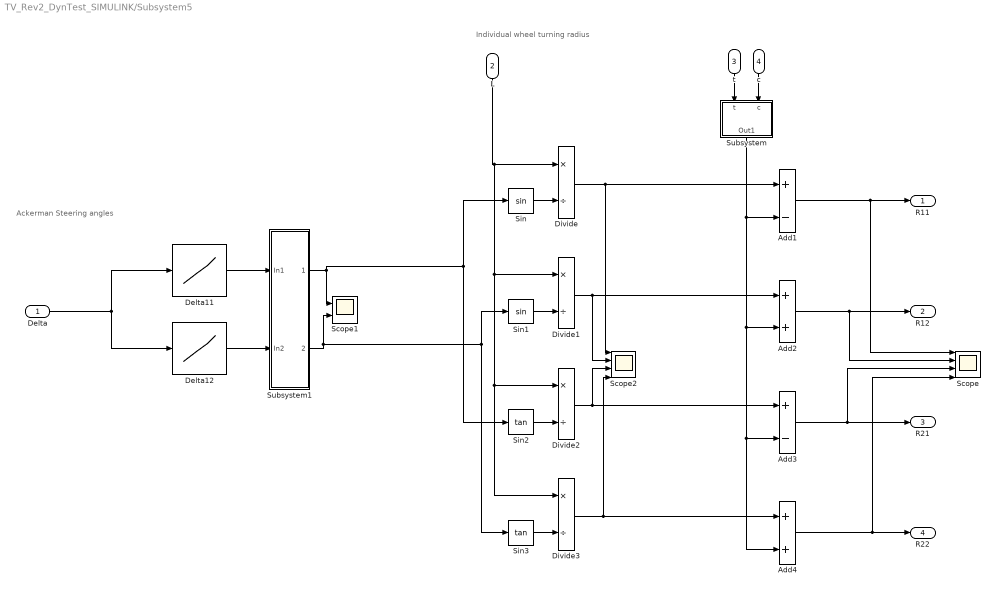
== system TV_Rev2_DynTest_SIMULINK/Subsystem5 ==
  note: Ackerman Steering angles
  note: Individual wheel turning radius
  Delta : Inport
  L : Inport  Port=2
  t : Inport  Port=3
  c : Inport  Port=4
  Add1 : Sum  Inputs=+-
  Add2 : Sum
  Add3 : Sum  Inputs=+-
  Add4 : Sum
  Delta11 : Lookup_n-D  NumberOfTableDimensions=1  BreakpointsForDimension1=DeltaT  BreakpointsForDimension1DataTypeStr=double  Table=Delta11T  TableDataTypeStr=double  InternalRulePriority=Speed  RndMeth=Simplest  InputSameDT=on
  Delta12 : Lookup_n-D  NumberOfTableDimensions=1  BreakpointsForDimension1=DeltaT  Table=Delta12T  TableDataTypeStr=Inherit: Inherit from 'Table data'  InternalRulePriority=Speed  RndMeth=Simplest  InputSameDT=on
  Divide{,1..3} (4 alike) : Product  Inputs=*/
  Scope : Scope  NumInputPorts=4
  Scope1 : Scope  NumInputPorts=2
  Scope2 : Scope  NumInputPorts=4
  Sin : Trigonometry
  Sin1 : Trigonometry
  Sin2 : Trigonometry  Operator=tan
  Sin3 : Trigonometry  Operator=tan
  Subsystem : Subsystem
  Subsystem1 : Subsystem
  R11 : Outport
  R12 : Outport  Port=2
  R21 : Outport  Port=3
  R22 : Outport  Port=4
  wires:
  Add1/1 -> Scope/1, R11/1
  Sin/1 -> Divide/2
  Divide/1 -> Add1/1, Scope2/1
  Divide1/1 -> Add2/1, Scope2/2
  Sin1/1 -> Divide1/2
  Add2/1 -> Scope/2, R12/1
  Divide2/1 -> Scope2/3, Add3/1
  Sin2/1 -> Divide2/2
  Subsystem/1(Out1) -> Add4/2, Add3/2, Add2/2, Add1/2
  Divide3/1 -> Scope2/4, Add4/1
  L/1 -> Divide3/1, Divide2/1, Divide1/1, Divide/1
  Sin3/1 -> Divide3/2
  Add4/1 -> Scope/4, R22/1
  Add3/1 -> Scope/3, R21/1
  Subsystem1/1(Delta11) -> Scope1/1, Sin2/1, Sin/1
  Subsystem1/2(Delta12) -> Sin3/1, Sin1/1, Scope1/2
  t/1 -> Subsystem/1(t)
  c/1 -> Subsystem/2(c)
  Delta12/1 -> Subsystem1/2(In2)
  Delta11/1 -> Subsystem1/1(In1)
  Delta/1 -> Delta11/1, Delta12/1

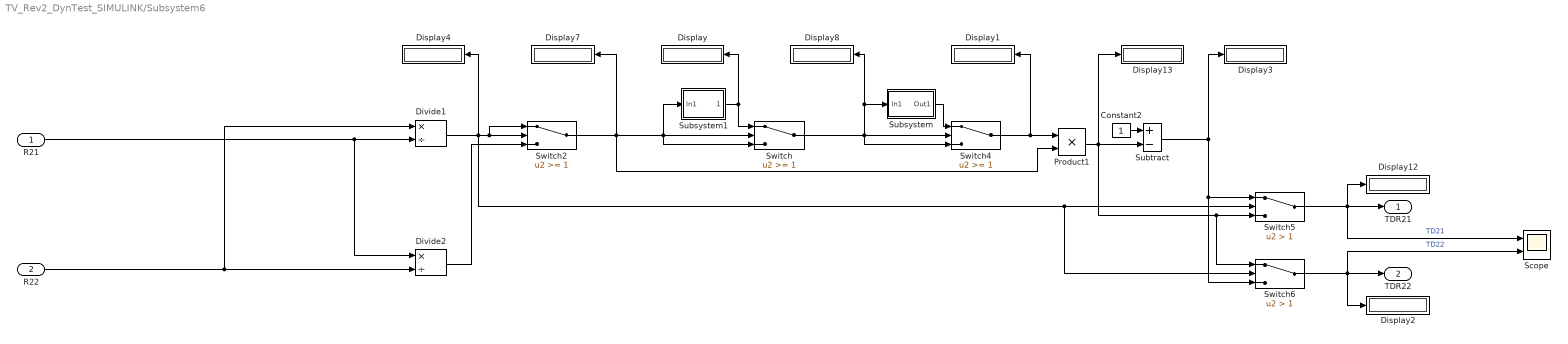
== system TV_Rev2_DynTest_SIMULINK/Subsystem6 ==
  R21 : Inport
  R22 : Inport  Port=2
  Constant2 : Constant
  Display{,1..4,7..8,12..13} (9 alike) : Display
  Divide1 : Product  Inputs=*/
  Divide2 : Product  Inputs=*/
  Product1 : Product
  Scope : Scope  NumInputPorts=2
  Subsystem : Subsystem
  Subsystem1 : Subsystem
  Subtract : Sum  Inputs=+-
  Switch : Switch  Threshold=1
  Switch2 : Switch  Threshold=1
  Switch4 : Switch  Threshold=1
  Switch5 : Switch  Criteria=u2 > Threshold  Threshold=1
  Switch6 : Switch  Criteria=u2 > Threshold  Threshold=1
  TDR21 : Outport
  TDR22 : Outport  Port=2
  wires:
  Switch6/1 -> Scope/2, Display2/1, TDR22/1  "TD22"
  R21/1 -> Divide2/1, Divide1/2
  Switch5/1 -> TDR21/1, Scope/1, Display12/1  "TD21"
  Subsystem/1(Out1) -> Switch4/1
  Switch/1 -> Switch4/3, Switch4/2, Display8/1, Subsystem/1(In1)
  Switch2/1 -> Product1/2, Display7/1, Switch/2, Switch/3, Subsystem1/1(In1)
  Subsystem1/1(Out1) -> Switch/1, Display/1
  Constant2/1 -> Subtract/1
  Subtract/1 -> Display3/1, Switch6/3, Switch5/1
  Product1/1 -> Switch6/1, Switch5/3, Display13/1, Subtract/2
  Divide2/1 -> Switch2/3
  Switch4/1 -> Product1/1, Display1/1
  Divide1/1 -> Switch6/2, Switch5/2, Display4/1, Switch2/1, Switch2/2
  R22/1 -> Divide1/1, Divide2/2

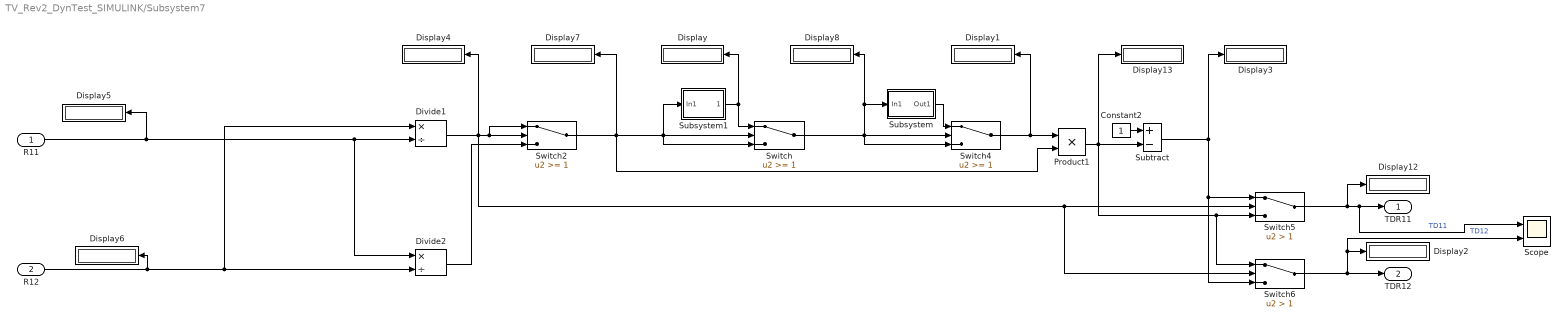
== system TV_Rev2_DynTest_SIMULINK/Subsystem7 ==
  R11 : Inport
  R12 : Inport  Port=2
  Constant2 : Constant
  Display{,1..8,12..13} (11 alike) : Display
  Divide1 : Product  Inputs=*/
  Divide2 : Product  Inputs=*/
  Product1 : Product
  Scope : Scope  NumInputPorts=2
  Subsystem : Subsystem
  Subsystem1 : Subsystem
  Subtract : Sum  Inputs=+-
  Switch : Switch  Threshold=1
  Switch2 : Switch  Threshold=1
  Switch4 : Switch  Threshold=1
  Switch5 : Switch  Criteria=u2 > Threshold  Threshold=1
  Switch6 : Switch  Criteria=u2 > Threshold  Threshold=1
  TDR11 : Outport
  TDR12 : Outport  Port=2
  wires:
  Switch6/1 -> Scope/2, Display2/1, TDR12/1  "TD12"
  R11/1 -> Display5/1, Divide2/1, Divide1/2
  Switch5/1 -> Display12/1, Scope/1, TDR11/1  "TD11"
  Subsystem/1(Out1) -> Switch4/1
  Switch/1 -> Switch4/3, Switch4/2, Display8/1, Subsystem/1(In1)
  Switch2/1 -> Product1/2, Display7/1, Switch/2, Switch/3, Subsystem1/1(In1)
  Subsystem1/1(Out1) -> Switch/1, Display/1
  Constant2/1 -> Subtract/1
  Subtract/1 -> Display3/1, Switch6/3, Switch5/1
  Product1/1 -> Switch6/1, Switch5/3, Display13/1, Subtract/2
  Divide2/1 -> Switch2/3
  Switch4/1 -> Product1/1, Display1/1
  Divide1/1 -> Switch6/2, Switch5/2, Display4/1, Switch2/1, Switch2/2
  R12/1 -> Display6/1, Divide1/1, Divide2/2

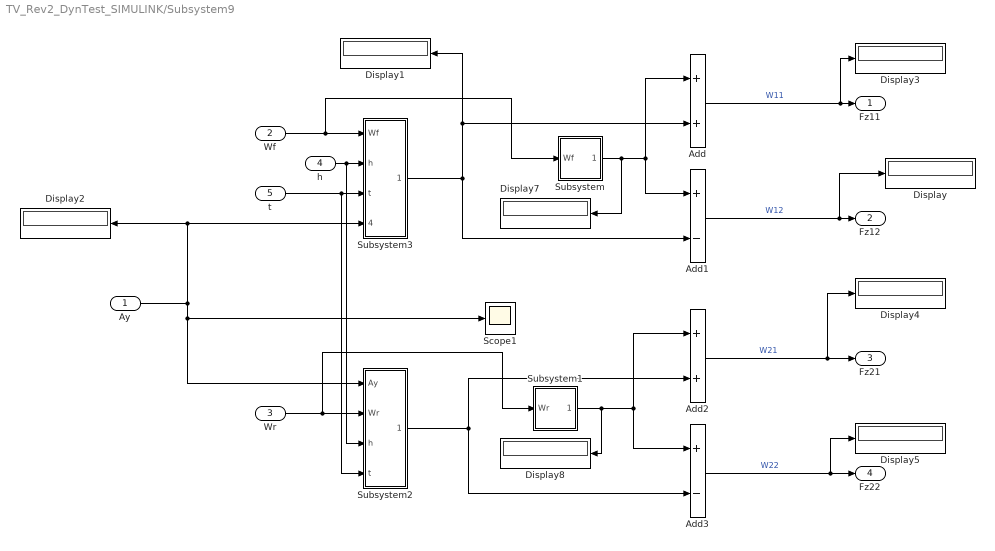
== system TV_Rev2_DynTest_SIMULINK/Subsystem9 ==
  Ay : Inport
  Wf : Inport  Port=2
  Wr : Inport  Port=3
  h : Inport  Port=4
  t : Inport  Port=5
  Add : Sum
  Add1 : Sum  Inputs=+-
  Add2 : Sum
  Add3 : Sum  Inputs=+-
  Display{,1..5,7..8} (8 alike) : Display
  Scope1 : Scope
  Subsystem : Subsystem
  Subsystem1 : Subsystem
  Subsystem2 : Subsystem
  Subsystem3 : Subsystem
  Fz11 : Outport
  Fz12 : Outport  Port=2
  Fz21 : Outport  Port=3
  Fz22 : Outport  Port=4
  wires:
  Add1/1 -> Display/1, Fz12/1  "W12"
  Subsystem1/1(Out1) -> Display8/1, Add2/1, Add3/1
  Add3/1 -> Display5/1, Fz22/1  "W22"
  Add/1 -> Display3/1, Fz11/1  "W11"
  Add2/1 -> Display4/1, Fz21/1  "W21"
  Ay/1 -> Display2/1, Subsystem3/4(In4), Scope1/1, Subsystem2/1(Ay)
  Subsystem/1(Out1) -> Display7/1, Add/1, Add1/1
  Wf/1 -> Subsystem3/1(Wf), Subsystem/1(Wf)
  Subsystem2/1(Out1) -> Add3/2, Add2/2
  Wr/1 -> Subsystem1/1(Wr), Subsystem2/2(Wr)
  h/1 -> Subsystem2/3(h), Subsystem3/2(h)
  t/1 -> Subsystem2/4(t), Subsystem3/3(t)
  Subsystem3/1(Out1) -> Add/2, Display1/1, Add1/2

== system TV_Rev2_DynTest_SIMULINK/TRatios scope1 ==
  TDR11 : Inport
  TDR12 : Inport  Port=2
  TDR21 : Inport  Port=3
  TDR22 : Inport  Port=4
  Add2 : Sum
  Add3 : Sum
  Ratios1 : Scope  NumInputPorts=2
  wires:
  Add3/1 -> Ratios1/2  "rear"
  TDR21/1 -> Add3/1
  Add2/1 -> Ratios1/1  "front"
  TDR12/1 -> Add2/2
  TDR22/1 -> Add3/2
  TDR11/1 -> Add2/1

== system TV_Rev2_DynTest_SIMULINK/TRatios scope2 ==
  TDR11 : Inport
  TDR12 : Inport  Port=2
  TDR21 : Inport  Port=3
  TDR22 : Inport  Port=4
  Add2 : Sum
  Add3 : Sum
  Ratios1 : Scope  NumInputPorts=2
  wires:
  TDR11/1 -> Add2/1
  TDR22/1 -> Add3/2
  TDR12/1 -> Add2/2
  Add2/1 -> Ratios1/1  "front"
  TDR21/1 -> Add3/1
  Add3/1 -> Ratios1/2  "rear"

== system TV_Rev2_DynTest_SIMULINK/TRatios scope3 ==
  TDR11 : Inport
  TDR12 : Inport  Port=2
  TDR21 : Inport  Port=3
  TDR22 : Inport  Port=4
  Add2 : Sum
  Add3 : Sum
  Ratios1 : Scope  NumInputPorts=2
  wires:
  TDR11/1 -> Add2/1
  TDR22/1 -> Add3/2
  TDR12/1 -> Add2/2
  Add2/1 -> Ratios1/1  "front"
  TDR21/1 -> Add3/1
  Add3/1 -> Ratios1/2  "rear"

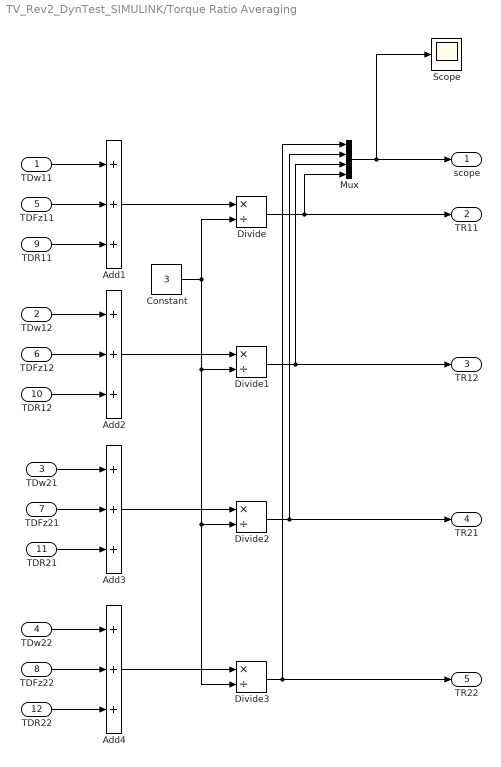
== system TV_Rev2_DynTest_SIMULINK/Torque Ratio Averaging ==
  TDw11 : Inport
  TDw12 : Inport  Port=2
  TDw21 : Inport  Port=3
  TDw22 : Inport  Port=4
  TDFz11 : Inport  Port=5
  TDFz12 : Inport  Port=6
  TDFz21 : Inport  Port=7
  TDFz22 : Inport  Port=8
  TDR11 : Inport  Port=9
  TDR12 : Inport  Port=10
  TDR21 : Inport  Port=11
  TDR22 : Inport  Port=12
  Add{1..4} (4 alike) : Sum  Inputs=+++
  Constant : Constant  Value=3
  Divide{,1..3} (4 alike) : Product  Inputs=*/
  Mux : Mux
  Scope : Scope
  scope : Outport
  TR11 : Outport  Port=2
  TR12 : Outport  Port=3
  TR21 : Outport  Port=4
  TR22 : Outport  Port=5
  wires:
  Divide2/1 -> Mux/2, TR21/1
  TDw21/1 -> Add3/1
  Add4/1 -> Divide3/1
  Divide3/1 -> Mux/1, TR22/1
  Divide1/1 -> Mux/3, TR12/1
  TDR11/1 -> Add1/3
  Add1/1 -> Divide/1
  Divide/1 -> Mux/4, TR11/1
  TDw22/1 -> Add4/1
  TDFz11/1 -> Add1/2
  Add3/1 -> Divide2/1
  Add2/1 -> Divide1/1
  TDFz12/1 -> Add2/2
  TDR12/1 -> Add2/3
  Constant/1 -> Divide/2, Divide3/2, Divide2/2, Divide1/2
  TDw11/1 -> Add1/1
  TDw12/1 -> Add2/1
  TDFz21/1 -> Add3/2
  TDR21/1 -> Add3/3
  TDR22/1 -> Add4/3
  TDFz22/1 -> Add4/2
  Mux/1 -> Scope/1, scope/1

== system TV_Rev2_DynTest_SIMULINK/Torque Ratios  ==
  In1 : Inport
  In2 : Inport  Port=2
  In3 : Inport  Port=3
  In4 : Inport  Port=4
  Add2 : Sum
  Add3 : Sum
  Ratios1 : Scope  NumInputPorts=2
  wires:
  Add3/1 -> Ratios1/2  "rear"
  In3/1 -> Add3/1
  Add2/1 -> Ratios1/1  "front"
  In2/1 -> Add2/2
  In4/1 -> Add3/2
  In1/1 -> Add2/1

== system TV_Rev2_DynTest_SIMULINK/Torque Variation ==
  In1 : Inport
  In2 : Inport  Port=2
  In3 : Inport  Port=3
  In4 : Inport  Port=4
  Add : Sum  Inputs=+-
  Add1 : Sum  Inputs=+-
  Scope : Scope
  Scope2 : Scope
  wires:
  Add/1 -> Scope/1
  In3/1 -> Add1/1
  In1/1 -> Add/1
  Add1/1 -> Scope2/1
  In4/1 -> Add1/2
  In2/1 -> Add/2

== system TV_Rev2_DynTest_SIMULINK/Subsystem10/Subsystem ==
  In1 : Inport
  Constant4 : Constant  Value=1/2
  Product : Product
  Out1 : Outport
  wires:
  In1/1 -> Product/2
  Product/1 -> Out1/1
  Constant4/1 -> Product/1

== system TV_Rev2_DynTest_SIMULINK/Subsystem10/Subsystem1 ==
  In1 : Inport
  Add : Sum
  Constant : Constant
  Divide2 : Product  Inputs=*/
  Out1 : Outport
  wires:
  In1/1 -> Add/1
  Add/1 -> Divide2/2
  Constant/1 -> Divide2/1, Add/2
  Divide2/1 -> Out1/1

== system TV_Rev2_DynTest_SIMULINK/Subsystem11/Subsystem ==
  In1 : Inport
  Constant4 : Constant  Value=1/2
  Product : Product
  Out1 : Outport
  wires:
  In1/1 -> Product/2
  Product/1 -> Out1/1
  Constant4/1 -> Product/1

== system TV_Rev2_DynTest_SIMULINK/Subsystem11/Subsystem1 ==
  In1 : Inport
  Add : Sum
  Constant : Constant
  Divide2 : Product  Inputs=*/
  Out1 : Outport
  wires:
  In1/1 -> Add/1
  Add/1 -> Divide2/2
  Constant/1 -> Divide2/1, Add/2
  Divide2/1 -> Out1/1

== system TV_Rev2_DynTest_SIMULINK/Subsystem2/Subsystem ==
  In1 : Inport
  Constant4 : Constant  Value=1/2
  Product : Product
  Out1 : Outport
  wires:
  Constant4/1 -> Product/1
  Product/1 -> Out1/1
  In1/1 -> Product/2

== system TV_Rev2_DynTest_SIMULINK/Subsystem2/Subsystem1 ==
  In1 : Inport
  Add : Sum
  Constant : Constant
  Divide2 : Product  Inputs=*/
  Out1 : Outport
  wires:
  Divide2/1 -> Out1/1
  Constant/1 -> Add/2, Divide2/1
  Add/1 -> Divide2/2
  In1/1 -> Add/1

== system TV_Rev2_DynTest_SIMULINK/Subsystem4/Subsystem ==
  In1 : Inport
  Constant4 : Constant  Value=1/2
  Product : Product
  Out1 : Outport
  wires:
  Constant4/1 -> Product/1
  Product/1 -> Out1/1
  In1/1 -> Product/2

== system TV_Rev2_DynTest_SIMULINK/Subsystem4/Subsystem1 ==
  In1 : Inport
  Add : Sum
  Constant : Constant
  Divide2 : Product  Inputs=*/
  Out1 : Outport
  wires:
  Divide2/1 -> Out1/1
  Constant/1 -> Add/2, Divide2/1
  Add/1 -> Divide2/2
  In1/1 -> Add/1

== system TV_Rev2_DynTest_SIMULINK/Subsystem5/Subsystem ==
  t : Inport
  c : Inport  Port=2
  Constant : Constant  Value=2
  Divide4 : Product  Inputs=*/
  Subtract : Sum  Inputs=+-
  Out1 : Outport
  wires:
  t/1 -> Subtract/1
  Divide4/1 -> Out1/1
  c/1 -> Subtract/2
  Subtract/1 -> Divide4/1
  Constant/1 -> Divide4/2

== system TV_Rev2_DynTest_SIMULINK/Subsystem5/Subsystem1 ==
  In1 : Inport
  In2 : Inport  Port=2
  Constant : Constant  Value=50
  Constant1 : Constant  Value=50
  Degrees to Radians : simulink_extras/Transformations/Degrees to Radians
  Degrees to Radians1 : simulink_extras/Transformations/Degrees to Radians
  Subtract : Sum  Inputs=+-
  Subtract1 : Sum  Inputs=+-
  Delta11 : Outport
  Delta12 : Outport  Port=2
  wires:
  Constant/1 -> Subtract/2
  In1/1 -> Subtract1/1
  Constant1/1 -> Subtract1/2
  In2/1 -> Subtract/1
  Subtract1/1 -> Degrees to Radians/1
  Subtract/1 -> Degrees to Radians1/1
  Degrees to Radians/1 -> Delta11/1
  Degrees to Radians1/1 -> Delta12/1

== system TV_Rev2_DynTest_SIMULINK/Subsystem6/Subsystem ==
  In1 : Inport
  Constant4 : Constant  Value=1/2
  Product : Product
  Out1 : Outport
  wires:
  In1/1 -> Product/2
  Product/1 -> Out1/1
  Constant4/1 -> Product/1

== system TV_Rev2_DynTest_SIMULINK/Subsystem6/Subsystem1 ==
  In1 : Inport
  Add : Sum
  Constant : Constant
  Divide2 : Product  Inputs=*/
  Out1 : Outport
  wires:
  In1/1 -> Add/1
  Add/1 -> Divide2/2
  Constant/1 -> Divide2/1, Add/2
  Divide2/1 -> Out1/1

== system TV_Rev2_DynTest_SIMULINK/Subsystem7/Subsystem ==
  In1 : Inport
  Constant4 : Constant  Value=1/2
  Product : Product
  Out1 : Outport
  wires:
  In1/1 -> Product/2
  Product/1 -> Out1/1
  Constant4/1 -> Product/1

== system TV_Rev2_DynTest_SIMULINK/Subsystem7/Subsystem1 ==
  In1 : Inport
  Add : Sum
  Constant : Constant
  Divide2 : Product  Inputs=*/
  Out1 : Outport
  wires:
  In1/1 -> Add/1
  Add/1 -> Divide2/2
  Constant/1 -> Divide2/1, Add/2
  Divide2/1 -> Out1/1

== system TV_Rev2_DynTest_SIMULINK/Subsystem9/Subsystem ==
  Wf : Inport
  Constant4 : Constant  Value=2
  Divide : Product  Inputs=*/
  Out1 : Outport
  wires:
  Constant4/1 -> Divide/2
  Divide/1 -> Out1/1
  Wf/1 -> Divide/1

== system TV_Rev2_DynTest_SIMULINK/Subsystem9/Subsystem1 ==
  Wr : Inport
  Constant4 : Constant  Value=2
  Divide : Product  Inputs=*/
  Out1 : Outport
  wires:
  Wr/1 -> Divide/1
  Divide/1 -> Out1/1
  Constant4/1 -> Divide/2

== system TV_Rev2_DynTest_SIMULINK/Subsystem9/Subsystem2 ==
  Ay : Inport
  Wr : Inport  Port=2
  h : Inport  Port=3
  t : Inport  Port=4
  Divide : Product  Inputs=*/
  Product : Product
  Product1 : Product
  Out1 : Outport
  wires:
  Ay/1 -> Product1/1
  Wr/1 -> Product1/2
  Product1/1 -> Product/2
  Product/1 -> Divide/1
  Divide/1 -> Out1/1
  h/1 -> Product/1
  t/1 -> Divide/2

== system TV_Rev2_DynTest_SIMULINK/Subsystem9/Subsystem3 ==
  Wf : Inport
  h : Inport  Port=2
  t : Inport  Port=3
  In4 : Inport  Port=4
  Divide : Product  Inputs=*/
  Product : Product
  Product1 : Product
  Out1 : Outport
  wires:
  Wf/1 -> Product1/1
  t/1 -> Divide/2
  h/1 -> Product1/2
  In4/1 -> Product/1
  Product1/1 -> Product/2
  Product/1 -> Divide/1
  Divide/1 -> Out1/1
